simulink model "Simulation3Draft_kush"  (R2023a)
settings: Solver=FixedStepDiscrete  StartTime=0.0  StopTime=180  FixedStep=0.01  RelTol=1e-3  EnableMultiTasking=on
undefined symbols (not defined in the file): InputPWM, ticksPerRot, wheelR, WheelSpeed
libraries: mobileRoboticsTrainingLib x7, slpidlib x2, commrandsrc3 x1
settings Model: ExtModeTrigDuration=2  Creator=Boitumelo  LastModifiedBy=ankus
settings SolverCC: AutoInsertRateTranBlk=on
settings OptimizationCC: EnhancedBackFolding=on  PassReuseOutputArgsAs=Individual arguments  ZeroExternalMemoryAtStartup=off  ZeroInternalMemoryAtStartup=off  MaxStackSize=64  OptimizeBlockOrder=speed  DifferentSizesBufferReuse=on  OptimizationCustomize=off  EfficientTunableParamExpr=on
settings DebuggingCC: ParameterTunabilityLossMsg=error  UnconnectedInputMsg=warning  UnconnectedOutputMsg=warning  UnconnectedLineMsg=warning
settings HardwareCC: ProdBitPerPointer=32  ProdBitPerSizeT=32  ProdBitPerPtrDiffT=32  ProdLargestAtomicInteger=Long  ProdLargestAtomicFloat=Double  ProdWordSize=32  ProdHWDeviceType=ARM Compatible->ARM Cortex  UseEmbeddedCoderFeatures=off
settings ModelReferenceCC: EnableRefExpFcnMdlSchedulingChecks=on
settings SFSimCC: MATLABDynamicMemAlloc=off
settings RTWCC: Description=Embedded Coder  SystemTargetFile=ert.tlc  HardwareBoard=Arduino Nano 33 IoT  TemplateMakefile=ert_default_tmf  Toolchain=Arduino ARM  BuildConfiguration=Faster Runs  DLArmComputeVersion=19.05
settings CodeAppCC: ForceParamTrailComments=on  IgnoreCustomStorageClasses=off  OperatorAnnotations=on  SimulinkDataObjDesc=on  SFDataObjDesc=on  InsertBlockDesc=on
settings ERTTargetCC: SupportContinuousTime=on  SupportNonInlinedSFcns=on  SupportVariableSizeSignals=on  ExtModeTransport=3  ExtModeStaticAlloc=on  ExtModeAutomaticAllocSize=off  ExtModeStaticAllocSize=8192  ExtModeMexFile=ext_xcp  ExtModeIntrfLevel=Level2 - Open

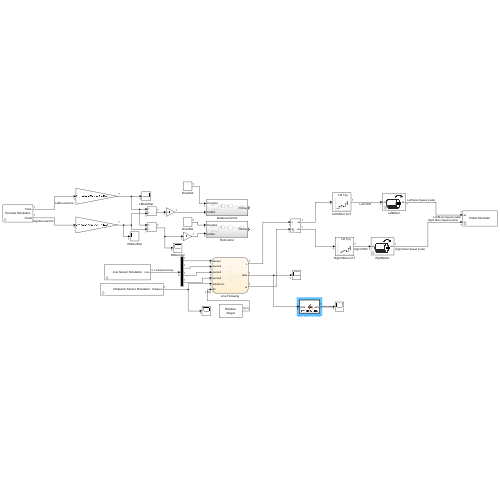
[thumbnail: Simulink's stored preview of the top-level diagram]
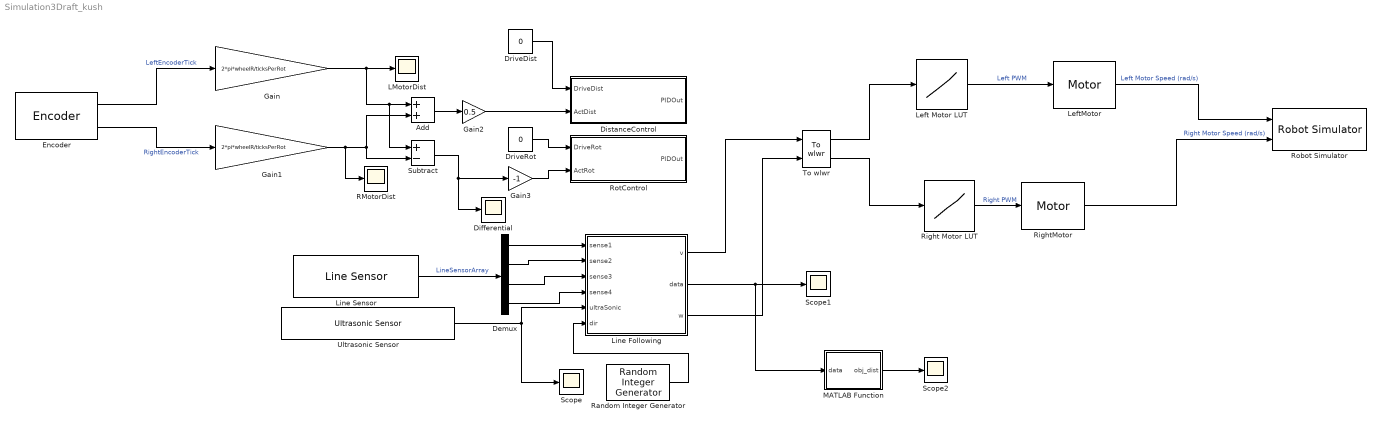
== system Simulation3Draft_kush ==
  Add : Sum
  Demux : Demux
  Differential : Scope
  DistanceControl : Subsystem
  DriveDist : Constant  Value=0
  DriveRot : Constant  Value=0
  Encoder : mobileRoboticsTrainingLib/Encoder  axleLength=axleLength  wheelR=wheelR  ticksPerRot=ticksPerRot
      settings: SourceProductName=Mobile Robotics Training Library
  Gain : Gain  Gain=2*pi*wheelR/ticksPerRot
  Gain1 : Gain  Gain=2*pi*wheelR/ticksPerRot
  Gain2 : Gain  Gain=0.5
  Gain3 : Gain  Gain=-1
  LMotorDist : Scope
  Left Motor LUT : Lookup_n-D  NumberOfTableDimensions=1  BreakpointsForDimension1=WheelSpeed  Table=InputPWM  InterpMethod=Nearest  ExtrapMethod=Clip  InternalRulePriority=Speed  RndMeth=Simplest
  LeftMotor : mobileRoboticsTrainingLib/Motor  motorPlant=wheelMotorModel  sensorType=Speed
      settings: SourceProductName=Mobile Robotics Training Library
  Line Following : Stateflow chart  TreatAsAtomicUnit=on
      settings: PortSchema="{\"entries\":[{\"content\":{\"sides\":[{\"content\":{\"connectorIds\":[\"In4\",\"In2\",\"In1\",\"In3\",\"In5\",\"In6\"]},\"type\":\"ConnectorPlacement.EquallySpacedRectSide\",\"uuid\":\"3c924089-815b-40f2-b705-e6f66b84a150\"},{\"content\":{\"connectorIds\":[\"Out1\",\"Out2\",\"Out3\"],\"side\":\"RIGHT\"},\"type\":\"ConnectorPlacement.EquallySpacedRectSide\",\"uuid\":\"d97906a3-7a34-4a96-a938-e8013b4137fd\"},{\"content\":{\"side\":\"TOP\"},\"type\":\"ConnectorPlacement.EquallySpacedRectSide\",\"uuid\":\"ab6da0b6-50e7-4a77-9ad9-89c802a4b943\"},{\"content\":{\"side\":\"BOTTOM\"},\"type\":\"ConnectorPlacement.EquallySpacedRectSide\",\"uuid\":\"37180fb4-5957-42f4-9c3a-063e4539371b\"}]},\"type\":\"ConnectorPlacement.EquallySpacedConnector\",\"uuid\":\"1e5cd3fb-bfdf-4f54-ace9-00fd0673d45b\"}],\"packageUris\":[\"http://schema.mathworks.com/mf0/Connector/R2020b\"],\"version\":\"1.0\"}"
  Line Sensor : mobileRoboticsTrainingLib/Line Sensor  mapVariable=mapForSim  envVal=1  lineVal=0  sensOff=[0.0643 0.0354; 0.0675 0.005; 0.0675 -0.005; 0.0643 -0.0354]
      settings: SourceProductName=Mobile Robotics Training Library
  MATLAB Function : MATLAB Function  TreatAsAtomicUnit=on
  RMotorDist : Scope
  Random Integer Generator : commrandsrc3/Random Integer Generator  SetSize=2  SeedSource=Auto  Seed=0  SampleTime=3  SamplesPerFrame=1  OutputDataType=boolean  SimulateUsing=Interpreted execution
  Right Motor LUT : Lookup_n-D  NumberOfTableDimensions=1  BreakpointsForDimension1=WheelSpeed  Table=InputPWM  InterpMethod=Nearest  ExtrapMethod=Clip  InternalRulePriority=Speed  RndMeth=Simplest
  RightMotor : mobileRoboticsTrainingLib/Motor  motorPlant=wheelMotorModel  sensorType=Speed
      settings: SourceProductName=Mobile Robotics Training Library
  Robot Simulator : mobileRoboticsTrainingLib/Robot Simulator  Priority=99  mapVar=mapForSim  startX=0.5  startY=1.4  startTheta=90  axleLength=axleLength  wheelR=wheelR
  RotControl : Subsystem
  Scope : Scope
  Scope1 : Scope
  Scope2 : Scope
  Subtract : Sum  Inputs=+-
  To wlwr : mobileRoboticsTrainingLib/To wlwr  axleLength=0.1  wheelR=0.05
      link override change parameters: Gain=[1 -axleLength/2; 1 axleLength/2]
  Ultrasonic Sensor : mobileRoboticsTrainingLib/Ultrasonic Sensor  mapVar=mapForSim  maxSenRange=0.3  minSenRange=0  senRes=0.01  sensOff=[0.0675 0]
      settings: SourceProductName=Mobile Robotics Training Library
  wires:
  Right Motor LUT/1 -> RightMotor/1  "Right PWM"
  Left Motor LUT/1 -> LeftMotor/1  "Left PWM"
  Encoder/1 -> Gain/1  "LeftEncoderTick"
  Encoder/2 -> Gain1/1  "RightEncoderTick"
  To wlwr/1 -> Left Motor LUT/1
  To wlwr/2 -> Right Motor LUT/1
  Line Sensor/1 -> Demux/1  "LineSensorArray"
  RightMotor/1 -> Robot Simulator/2  "Right Motor Speed (rad/s)"
  LeftMotor/1 -> Robot Simulator/1  "Left Motor Speed (rad/s)"
  Gain/1 -> Subtract/1, Add/1, LMotorDist/1
  Gain1/1 -> RMotorDist/1, Subtract/2, Add/2
  Add/1 -> Gain2/1
  DriveDist/1 -> DistanceControl/1(DriveDist)
  Gain2/1 -> DistanceControl/2(ActDist)
  DriveRot/1 -> RotControl/1(DriveRot)
  Subtract/1 -> Gain3/1, Differential/1
  Demux/1 -> Line Following/4(sense1)
  Demux/2 -> Line Following/2(sense2)
  Demux/3 -> Line Following/1(sense3)
  Demux/4 -> Line Following/3(sense4)
  Gain3/1 -> RotControl/2(ActRot)
  Line Following/3(w) -> To wlwr/2
  Line Following/1(v) -> To wlwr/1
  Ultrasonic Sensor/1 -> Scope/1, Line Following/5(ultraSonic)
  Line Following/2(data) -> MATLAB Function/1(data), Scope1/1
  Random Integer Generator/1 -> Line Following/6(dir)
  MATLAB Function/1(obj_dist) -> Scope2/1

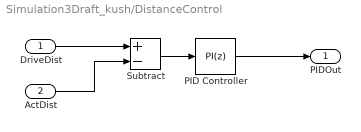
== system Simulation3Draft_kush/DistanceControl ==
  DriveDist : Inport
  ActDist : Inport  Port=2
  PID Controller : slpidlib/PID Controller  Controller=PI  Form=Parallel  TimeDomain=Discrete-time  UseExternalTs=off  SampleTime=-1  IntegratorMethod=Forward Euler  FilterMethod=Forward Euler  ControllerParametersSource=internal  P=5  I=1  UseKiTs=off  D=-1.16127933457653  N=26.3656587164613  UseFilter=on  TunerSelectOption=Transfer Function Based (PID Tuner App)  InitialConditionSource=internal  InitialConditionForIntegrator=0  InitialConditionForFilter=0  DifferentiatorICPrevScaledInput=0  ExternalReset=none  TrackingMode=off  Kt=1  LimitOutput=on  SatLimitsSource=internal  UpperSaturationLimit=0.67  LowerSaturationLimit=-0.67  LinearizeAsGain=on  AntiWindupMode=clamping  Kb=1  LimitIntegrator=off  UpperIntegratorSaturationLimit=inf  LowerIntegratorSaturationLimit=-inf  POutMin=[]  POutMax=[]  IOutMin=[]  IOutMax=[]  DOutMin=[]  DOutMax=[]  NOutMin=[]  NOutMax=[]  SumOutMin=[]  SumOutMax=[]  SaturationOutMin=[]  SaturationOutMax=[]  PParamMin=[]  PParamMax=[]  IParamMin=[]  IParamMax=[]  DParamMin=[]  DParamMax=[]  NParamMin=[]  NParamMax=[]  KbParamMin=[]  KbParamMax=[]  KtParamMin=[]  KtParamMax=[]  KbOutMin=[]  KbOutMax=[]  KtOutMin=[]  KtOutMax=[]  IntegratorOutMin=[]  IntegratorOutMax=[]  FilterOutMin=[]  FilterOutMax=[]  SumI1OutMin=[]  SumI1OutMax=[]  SumI2OutMin=[]  SumI2OutMax=[]  SumI3OutMin=[]  SumI3OutMax=[]  SumI4OutMin=[]  SumI4OutMax=[]  SumDOutMin=[]  SumDOutMax=[]  DifferentiatorOutMin=[]  DifferentiatorOutMax=[]  FilterDiffOutCoefMin=[]  FilterDiffOutCoefMax=[]  ReciprocalOutMin=[]  ReciprocalOutMax=[]  SumDenOutMin=[]  SumDenOutMax=[]  SumNumOutMin=[]  SumNumOutMax=[]  DivideOutMin=[]  DivideOutMax=[]  UdiffTsProdOutMin=[]  UdiffTsProdOutMax=[]  NTsProdOutMin=[]  NTsProdOutMax=[]  UintegralTsProdOutMin=[]  UintegralTsProdOutMax=[]  UngainTsProdOutMin=[]  UngainTsProdOutMax=[]  ClampingZeroOutDataTypeStr=Inherit: Inherit via back propagation  ClampingZeroOutMin=[]  ClampingZeroOutMax=[]  FilterDenConstantOutDataTypeStr=Inherit: Inherit via back propagation  FilterDenConstantOutMin=[]  FilterDenConstantOutMax=[]  PCopyOutDataTypeStr=Inherit: Inherit via back propagation  PCopyOutMin=[]  PCopyOutMax=[]  NCopyOutDataTypeStr=Inherit: Inherit via back propagation  NCopyOutMin=[]  NCopyOutMax=[]  IntegratorContinuousStateAttributes=''  IntegratorStateMustResolveToSignalObject=off  IntegratorRTWStateStorageClass=Auto  FilterContinuousStateAttributes=''  FilterStateMustResolveToSignalObject=off  FilterRTWStateStorageClass=Auto  ParallelPVariant=InternalParameters  IdealPVariant=Disabled  IVariant=InternalParameters  DVariant=Disabled  IntegratorVariant=Discrete  SatVariant=Enabled  AWVariant=DiscClampingParallel  PCopyVariant=Disabled  TRVariant=Disabled  FdbkBlocksVariant=Forward  IdealPFdbkVariant=Disabled  SatFdbkVariant=Disabled  DerivativeFilterVariant=Disabled  NVariant=Disabled  NCopyVariant=Disabled_SignalSpec  FilterICVariant=Disabled  IntegratorICVariant=InternalICs  ExternalResetVariant=Disabled  TRSumVariant=Passthrough  SumFdbkVariant=Disabled  SumVariant=Sum_PI  TsampFilterVariant=InternalTs  TsampNgainVariant=Passthrough  TsampIntegralVariant=Disabled_SignalSpec  ExternalSaturationOutDataTypeStr=Inherit: Same as second input
  Subtract : Sum  Inputs=+-
  PIDOut : Outport
  wires:
  DriveDist/1 -> Subtract/1
  ActDist/1 -> Subtract/2
  PID Controller/1 -> PIDOut/1
  Subtract/1 -> PID Controller/1

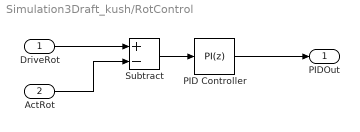
== system Simulation3Draft_kush/RotControl ==
  DriveRot : Inport
  ActRot : Inport  Port=2
  PID Controller : slpidlib/PID Controller  Controller=PI  Form=Parallel  TimeDomain=Discrete-time  UseExternalTs=off  SampleTime=-1  IntegratorMethod=Forward Euler  FilterMethod=Forward Euler  ControllerParametersSource=internal  P=20  I=10  UseKiTs=off  D=0  N=100  UseFilter=on  TunerSelectOption=Transfer Function Based (PID Tuner App)  InitialConditionSource=internal  InitialConditionForIntegrator=0  InitialConditionForFilter=0  DifferentiatorICPrevScaledInput=0  ExternalReset=none  TrackingMode=off  Kt=1  LimitOutput=on  SatLimitsSource=internal  UpperSaturationLimit=0.67  LowerSaturationLimit=-0.67  LinearizeAsGain=on  AntiWindupMode=clamping  Kb=1  LimitIntegrator=off  UpperIntegratorSaturationLimit=inf  LowerIntegratorSaturationLimit=-inf  POutMin=[]  POutMax=[]  IOutMin=[]  IOutMax=[]  DOutMin=[]  DOutMax=[]  NOutMin=[]  NOutMax=[]  SumOutMin=[]  SumOutMax=[]  SaturationOutMin=[]  SaturationOutMax=[]  PParamMin=[]  PParamMax=[]  IParamMin=[]  IParamMax=[]  DParamMin=[]  DParamMax=[]  NParamMin=[]  NParamMax=[]  KbParamMin=[]  KbParamMax=[]  KtParamMin=[]  KtParamMax=[]  KbOutMin=[]  KbOutMax=[]  KtOutMin=[]  KtOutMax=[]  IntegratorOutMin=[]  IntegratorOutMax=[]  FilterOutMin=[]  FilterOutMax=[]  SumI1OutMin=[]  SumI1OutMax=[]  SumI2OutMin=[]  SumI2OutMax=[]  SumI3OutMin=[]  SumI3OutMax=[]  SumI4OutMin=[]  SumI4OutMax=[]  SumDOutMin=[]  SumDOutMax=[]  DifferentiatorOutMin=[]  DifferentiatorOutMax=[]  FilterDiffOutCoefMin=[]  FilterDiffOutCoefMax=[]  ReciprocalOutMin=[]  ReciprocalOutMax=[]  SumDenOutMin=[]  SumDenOutMax=[]  SumNumOutMin=[]  SumNumOutMax=[]  DivideOutMin=[]  DivideOutMax=[]  UdiffTsProdOutMin=[]  UdiffTsProdOutMax=[]  NTsProdOutMin=[]  NTsProdOutMax=[]  UintegralTsProdOutMin=[]  UintegralTsProdOutMax=[]  UngainTsProdOutMin=[]  UngainTsProdOutMax=[]  ClampingZeroOutDataTypeStr=Inherit: Inherit via back propagation  ClampingZeroOutMin=[]  ClampingZeroOutMax=[]  FilterDenConstantOutDataTypeStr=Inherit: Inherit via back propagation  FilterDenConstantOutMin=[]  FilterDenConstantOutMax=[]  PCopyOutDataTypeStr=Inherit: Inherit via back propagation  PCopyOutMin=[]  PCopyOutMax=[]  NCopyOutDataTypeStr=Inherit: Inherit via back propagation  NCopyOutMin=[]  NCopyOutMax=[]  IntegratorContinuousStateAttributes=''  IntegratorStateMustResolveToSignalObject=off  IntegratorRTWStateStorageClass=Auto  FilterContinuousStateAttributes=''  FilterStateMustResolveToSignalObject=off  FilterRTWStateStorageClass=Auto  ParallelPVariant=InternalParameters  IdealPVariant=Disabled  IVariant=InternalParameters  DVariant=Disabled  IntegratorVariant=Discrete  SatVariant=Enabled  AWVariant=DiscClampingParallel  PCopyVariant=Disabled  TRVariant=Disabled  FdbkBlocksVariant=Forward  IdealPFdbkVariant=Disabled  SatFdbkVariant=Disabled  DerivativeFilterVariant=Disabled  NVariant=Disabled  NCopyVariant=Disabled_SignalSpec  FilterICVariant=Disabled  IntegratorICVariant=InternalICs  ExternalResetVariant=Disabled  TRSumVariant=Passthrough  SumFdbkVariant=Disabled  SumVariant=Sum_PI  TsampFilterVariant=InternalTs  TsampNgainVariant=Passthrough  TsampIntegralVariant=Disabled_SignalSpec  ExternalSaturationOutDataTypeStr=Inherit: Same as second input
  Subtract : Sum  Inputs=+-
  PIDOut : Outport
  wires:
  DriveRot/1 -> Subtract/1
  ActRot/1 -> Subtract/2
  PID Controller/1 -> PIDOut/1
  Subtract/1 -> PID Controller/1

== stateflow chart Simulation3Draft_kush/Line Following ==
  state Random
    entry:
    dir;
  state notEnd
    entry:
    v=-0.05;
  state End
    entry:
    v=0;
    w=0;
  state checkEnd
    entry:
    v=0.05;
  state TurnLeft
    entry:
    v=0.01;
    w=0.4;
  state TurnRight
    entry:
    v=0.01;
    w=-0.4;
  state Drive
    entry:
    v=0.05;
    w=0;
    i=0;
  state CorrectRight
    entry:
    v=0.01;
    w=-0.8
  state CorrectLeft
    entry:
    v=0.01;
    w=0.8
  state ObjectDetected
    entry:
    v=0.1;
    i=1;
  state CorrectRight1
    entry:
    w=-0.5
  state CorrectLeft1
    entry:
    w=0.5
  state EndOfLine
    entry:
    v=0;
  state TurnAround1
    entry:
    data=ultraSonic;
    w=0.6;
    exit:
    ultraSonic;
  Random -> TurnLeft [order 2] : [dir==1]
  Random -> TurnRight [order 1] : [dir==0]
  notEnd -> Random : [after(0.5,sec)]
  checkEnd -> notEnd [order 1] : [after(0.5,sec) &&sense1 == 1 && sense2 == 1 && sense3 ==1 && sense4==1 ]
  checkEnd -> End [order 2] : [after(0.5,sec) &&sense1 ==0 && sense2 == 0 && sense3 ==0 && sense4==0 ]
  Drive -> checkEnd [order 1] : [sense1 == 0 && sense2 == 0 && sense3 == 0 && sense4==0]
  (default) -> Drive
  TurnRight -> Drive : [after(0.5,sec) && sense2 ==0 && sense3 ==0]
  Drive -> TurnLeft [order 6] : [after(0.5,sec) && sense2 == 0 && sense3 == 0 && sense1 == 0 ]
  TurnLeft -> Drive : [sense2==0 && sense3==0 && after(0.5,sec)]
  Drive -> TurnRight [order 3] : [after(0.5,sec) && sense2 == 0 && sense3 == 0 && sense4 == 0 && sense1==1]
  Drive -> CorrectRight [order 2] : [sense2==1 && sense3 ==0 && sense1 == 1 &&sense4 ==1]
  Drive -> CorrectLeft [order 4] : [sense2==0 && sense3 ==1 && sense1 == 1 &&sense4 ==1]
  CorrectRight -> Drive : [sense2==0 && sense3 == 0]
  CorrectLeft -> Drive : [sense2 ==0 && sense3 ==0]
  TurnAround1 -> Drive : [after(1,sec) && sense2 == 0 && sense3 == 0]
  Drive -> EndOfLine [order 7] : [sense1 == 1 && sense2 == 1 && sense3 == 1 && sense4==1]
  Drive -> ObjectDetected [order 5] : [ultraSonic ~= 0]
  ObjectDetected -> CorrectRight1 [order 2] : [sense2==1 && sense3 ==0]
  ObjectDetected -> CorrectLeft1 [order 3] : [sense2==0 && sense3 ==1]
  CorrectRight1 -> ObjectDetected : [sense2==0 && sense3 == 0]
  CorrectLeft1 -> ObjectDetected : [sense2 ==0 && sense3 ==0]
  ObjectDetected -> EndOfLine [order 1] : [sense1 == 0 && sense4 == 0]
  EndOfLine -> TurnAround1 : [after(1,sec)]
  data: v output; data output; w output; sense3 input; sense2 input; sense4 input; sense1 input; ultraSonic input; i local; dir input

== matlab function Simulation3Draft_kush/MATLAB Function ==
  data: data input; obj_dist output [0..10]
function obj_dist = dynamicArray(data)

    persistent obj_dist_array;
    
    if isempty(obj_dist_array)
        obj_dist_array = [];
    end
    
    % Add data to the array
    obj_dist_array = [obj_dist_array, data];
    
    % Output the array
    obj_dist = obj_dist_array;

end
